simulink model "MC_Phase2_Part2_Q1"  (R2020b)
settings: Solver=VariableStepAuto  StartTime=0.0  StopTime=10.0  RelTol=1e-3
settings Model: Creator=ASUS  LastModifiedBy=ASUS

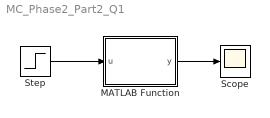
== system MC_Phase2_Part2_Q1 ==
  MATLAB Function : MATLAB Function  TreatAsAtomicUnit=on
  Scope : Scope
  Step : Step  Time=0  After=0.5*4096  SampleTime=0
  wires:
  Step/1 -> MATLAB Function/1(u)
  MATLAB Function/1(y) -> Scope/1

== matlab function MC_Phase2_Part2_Q1/MATLAB Function ==
  data: u input; y output
function y = fcn(u)
temp = -u / (4096*4) ;
temp = temp*(2*pi) ;
temp = temp - pi ;                         % Start point

while 1                                    % Set teta between -pi and +pi
    if (temp >= -pi)&&(temp <= pi)
        break
    end
    if temp < -pi
        temp = temp + 2*pi ;
    end
    if temp > pi
        temp = temp - 2*pi ;
    end
end

if (temp >= -pi)&&(temp <= (-pi/2))        % 3 ----> 1
    temp = temp + pi ;
end
if (temp >= (pi/2))&&(temp <= pi)          % 4 ----> 2
    temp = temp - pi ;
end

y = temp ;
